simulink model "pv_and_wind_completed"  (R2018a)
settings: Solver=VariableStepAuto  StartTime=0.0  StopTime=2.4  RelTol=1e-3
libraries: powerlib x50, powerlib_meascontrol x12, simulink x10, re_lib x2, peGeneralControl x1, simulink_extras x1
(part 1 of 2)
settings SolverCC: AlgebraicLoopSolver=LineSearch

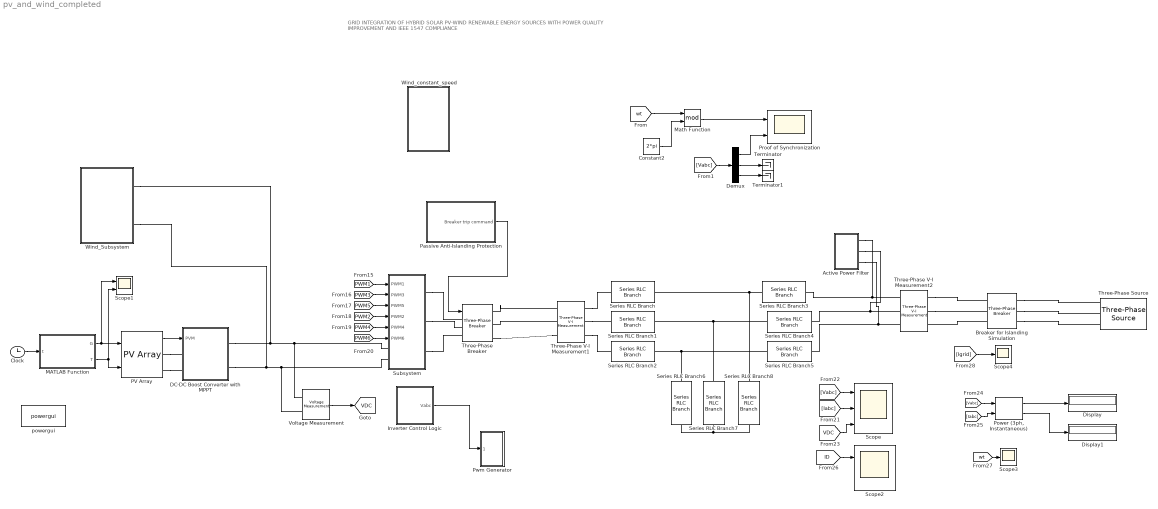
== system pv_and_wind_completed ==
  note: GRID INTEGRATION OF HYBRID SOLAR PV-WIND RENEWABLE ENERGY SOURCES WITH POWER QUALITY IMPROVEMENT AND IEEE 1547 COMPLIANCE
  Active Power Filter : Subsystem
  Breaker for Islanding Simulation : powerlib/Elements/Three-Phase Breaker  InitialState=closed  SwitchA=on  SwitchB=on  SwitchC=on  SwitchTimes=[9999]  External=off  BreakerResistance=0.01  SnubberResistance=1e6  SnubberCapacitance=inf  Measurements=None
  Clock : Clock
  Constant2 : Constant  Value=2*pi
  DC-DC Boost Converter with MPPT : Subsystem
  Demux : Demux  Outputs=3
  Display : Display
  Display1 : Display
  Inverter Control Logic : Subsystem
  MATLAB Function : MATLAB Function  TreatAsAtomicUnit=on
  Math Function : Math  Operator=mod  SaturateOnIntegerOverflow=on
  PV Array : re_lib/Solar/PV Array  Npar=40  Nser=10  PlotType=array @ 1000 W/m2 & specified temperatures  S_vec="[ 1000  500  100 ]"  Temp_C_vec="[ 45 25  ]"  ModuleName=1Soltech 1STH-215-P  PlotWhenSelected=off  Pm=213.15  Ncell=60  Voc=36.3  Isc=7.84  Vm=29  Im=7.35  beta_Voc_pc=-0.36099  alpha_Isc_pc=0.102  beta_Voc=-0.13104  alpha_Isc=0.007997  IL=7.8649  I0=2.9259e-10  nI=0.98117  Rsh=313.3991  Rs=0.39383  BAL=off  Tc=1e-6  Tfilter=5e-5
  Passive Anti-Islanding Protection : Subsystem
  "Power (3ph, Instantaneous)" : powerlib_meascontrol/Measurements/Power (3ph, Instantaneous)
      settings: SourceProductName=Simscape Power Systems
  Proof of Synchronization : Scope  NumInputPorts=2
  "Pwm Generator " : Subsystem
  Scope : Scope  NumInputPorts=3
  Scope1 : Scope  NumInputPorts=2
  Scope2 : Scope  NumInputPorts=2
  Scope3 : Scope
  Scope4 : Scope
  Series RLC Branch : powerlib/Elements/Series RLC Branch  LConnTagsString=__new0  RConnTagsString=__new0  BranchType=RL  Resistance=1e-3  Inductance=1e-3  SetiL0=off  InitialCurrent=0  Capacitance=1e-6  Setx0=off  InitialVoltage=0  Measurements=None
  Series RLC Branch1 : powerlib/Elements/Series RLC Branch  LConnTagsString=__new0  RConnTagsString=__new0  BranchType=RL  Resistance=1e-3  Inductance=1e-3  SetiL0=off  InitialCurrent=0  Capacitance=1e-6  Setx0=off  InitialVoltage=0  Measurements=None
  Series RLC Branch2 : powerlib/Elements/Series RLC Branch  LConnTagsString=__new0  RConnTagsString=__new0  BranchType=RL  Resistance=1e-3  Inductance=1e-3  SetiL0=off  InitialCurrent=0  Capacitance=1e-6  Setx0=off  InitialVoltage=0  Measurements=None
  Series RLC Branch3 : powerlib/Elements/Series RLC Branch  LConnTagsString=__new0  RConnTagsString=__new0  BranchType=RL  Resistance=1e-3  Inductance=0.5e-3  SetiL0=on  InitialCurrent=10  Capacitance=1e-6  Setx0=off  InitialVoltage=0  Measurements=None
  Series RLC Branch4 : powerlib/Elements/Series RLC Branch  LConnTagsString=__new0  RConnTagsString=__new0  BranchType=RL  Resistance=1e-3  Inductance=0.5e-3  SetiL0=on  InitialCurrent=10  Capacitance=1e-6  Setx0=off  InitialVoltage=0  Measurements=None
  Series RLC Branch5 : powerlib/Elements/Series RLC Branch  LConnTagsString=__new0  RConnTagsString=__new0  BranchType=RL  Resistance=1e-3  Inductance=0.5e-3  SetiL0=on  InitialCurrent=10  Capacitance=1e-6  Setx0=off  InitialVoltage=0  Measurements=None
  Series RLC Branch6 : powerlib/Elements/Series RLC Branch  LConnTagsString=__new0  RConnTagsString=__new0  BranchType=RC  Resistance=1e-3  Inductance=1000e-3  SetiL0=off  InitialCurrent=0  Capacitance=100e-6  Setx0=off  InitialVoltage=0  Measurements=None
  Series RLC Branch7 : powerlib/Elements/Series RLC Branch  LConnTagsString=__new0  RConnTagsString=__new0  BranchType=RC  Resistance=1e-3  Inductance=1000e-3  SetiL0=off  InitialCurrent=0  Capacitance=100e-6  Setx0=off  InitialVoltage=0  Measurements=None
  Series RLC Branch8 : powerlib/Elements/Series RLC Branch  LConnTagsString=__new0  RConnTagsString=__new0  BranchType=RC  Resistance=1e-3  Inductance=1000e-3  SetiL0=off  InitialCurrent=0  Capacitance=100e-6  Setx0=off  InitialVoltage=0  Measurements=None
  Subsystem : Subsystem
  Terminator : Terminator
  Terminator1 : Terminator
  Three-Phase V-I Measurement1 : powerlib/Measurements/Three-Phase V-I Measurement  VoltageMeasurement=no  SetLabelV=off  LabelV=Vabc  Vpu=off  VpuLL=off  CurrentMeasurement=yes  SetLabelI=on  LabelI=Iabc  Ipu=off  Pbase=100e6  Vbase=500e3  OutputType=Complex  PhasorSimulation=off  PSBequivalent=0
  Three-Phase V-I Measurement2 : powerlib/Measurements/Three-Phase V-I Measurement  VoltageMeasurement=phase-to-ground  SetLabelV=on  LabelV=Vabc  Vpu=off  VpuLL=off  CurrentMeasurement=yes  SetLabelI=on  LabelI=Igrid  Ipu=off  Pbase=100e6  Vbase=500e3  OutputType=Complex  PhasorSimulation=off  PSBequivalent=0
  Three-Phase Breaker : powerlib/Elements/Three-Phase Breaker  InitialState=closed  SwitchA=on  SwitchB=on  SwitchC=on  SwitchTimes=[9999]  External=on  BreakerResistance=0.01  SnubberResistance=1e6  SnubberCapacitance=inf  Measurements=None
  Three-Phase Source : powerlib/Electrical Sources/Three-Phase Source  InternalConnection=Yg  VoltagePhases=off  Voltage=400  PhaseAngle=0  Voltage_phases=[25e3 25e3 25e3]/sqrt(3)  PhaseAngles_phases=[0 -120 +120]  Frequency=50  NonIdealSource=on  SpecifyImpedance=off  Resistance=1e-3  Inductance=1e-5  ShortCircuitLevel=10e-6  BaseVoltage=400  XRratio=7  BusType=swing  Pref=10e3  Qref=0  Prefabc=[10e3, 10e3, 10e3]  Qrefabc=[0, 0, 0]  Qmin=-inf  Qmax=inf
  Voltage Measurement : powerlib/Measurements/Voltage Measurement  PhasorSimulation=off  OutputType=Complex  PSBequivalent=0
  Wind_Subsystem : Subsystem
  "Wind_constant_speed " : Subsystem
  powergui : powerlib/powergui  Priority=1  SimulationMode=Discrete  SampleTime=1e-6  frequency=60  Iterations=50  frequencyindice=0  Pbase=100e6  ErrMax=1e-4  UnitsV=kV  UnitsW=MW  buscounter=0  FunctionMessages=off  echomessages=off  EnableUseOfTLC=off  CurrentSourceSwitches=off  DisableSnubberDevices=off  DisableRonSwitches=off  DisableVfSwitches=off  DisplayEquations=off  SolverType=Tustin/Backward Euler (TBE)  Interpol=off  ExternalGateDelay=off  methode=off  Ts=100  x0status=blocks  SPID=off  SwTol=0  HookPort=off  RestoreLinks=warning  ResistiveCurrentMeasurement=off  Frange=[0:2:500]  Ylog=off  Xlog=on  ShowGrid=off  save=off  variable=ZData  structure=Grid_current  ZoomFFT=off  StartTime=0.4  cycles=5  DisplayStyle=1  fundamental=50  FreqAxis=off  MaxFrequency=1000  frequencyindicesteady=1  RmsSteady=1  display=off
  tag scope: VDC=global
  wires:
  Voltage Measurement/1 -> [VDC]
  [PWM6] -> Subsystem/6(PWM6)
  [PWM1] -> Subsystem/1(PWM1)
  "Power (3ph, Instantaneous)"/1 -> Display/1
  PV Array/1 -> DC-DC Boost Converter with MPPT/1("PVM ")
  [Iabc] -> "Power (3ph, Instantaneous)"/2
  [PWM3] -> Subsystem/2(PWM3)
  [Igrid] -> Scope4/1
  Inverter Control Logic/1(Vabc) -> "Pwm Generator "/1(1)
  [PWM4] -> Subsystem/5(PWM4)
  [Vabc] -> Scope/1
  [Vabc] -> "Power (3ph, Instantaneous)"/1
  [ID] -> Scope2/1
  "Power (3ph, Instantaneous)"/2 -> Display1/1
  [wt] -> Scope3/1
  [PWM2] -> Subsystem/4(PWM2)
  [VDC] -> Scope/3
  [PWM5] -> Subsystem/3(PWM5)
  [Iabc] -> Scope/2
  Passive Anti-Islanding Protection/1("Breaker trip command ") -> Three-Phase Breaker/1
  Demux/1 -> Proof of Synchronization/2
  Demux/2 -> Terminator/1
  Constant2/1 -> Math Function/2
  [wt] -> Math Function/1
  Math Function/1 -> Proof of Synchronization/1
  [Vabc] -> Demux/1
  Demux/3 -> Terminator1/1
  MATLAB Function/1(G) -> Scope1/1, PV Array/1
  MATLAB Function/2(T) -> Scope1/2, PV Array/2
  Clock/1 -> MATLAB Function/1(t)
  connections:
  Series RLC Branch7/RConn1 -- Series RLC Branch8/RConn1 -- Series RLC Branch6/RConn1
  Series RLC Branch8/LConn1 -- Series RLC Branch/RConn1 -- Series RLC Branch3/LConn1
  Series RLC Branch7/LConn1 -- Series RLC Branch1/RConn1 -- Series RLC Branch4/LConn1
  Series RLC Branch6/LConn1 -- Series RLC Branch2/RConn1 -- Series RLC Branch5/LConn1
  PV Array/RConn1 -- DC-DC Boost Converter with MPPT/LConn1
  Series RLC Branch3/RConn1 -- Active Power Filter/RConn1 -- Three-Phase V-I Measurement2/RConn1
  Series RLC Branch4/RConn1 -- Active Power Filter/RConn2 -- Three-Phase V-I Measurement2/RConn2
  Three-Phase V-I Measurement1/RConn3 -- Series RLC Branch2/LConn1
  Three-Phase V-I Measurement1/RConn1 -- Series RLC Branch/LConn1
  PV Array/RConn2 -- DC-DC Boost Converter with MPPT/LConn2
  Three-Phase V-I Measurement1/RConn2 -- Series RLC Branch1/LConn1
  Series RLC Branch5/RConn1 -- Active Power Filter/RConn3 -- Three-Phase V-I Measurement2/RConn3
  DC-DC Boost Converter with MPPT/RConn1 -- Wind_Subsystem/RConn1 -- Subsystem/LConn1 -- Voltage Measurement/LConn1
  DC-DC Boost Converter with MPPT/RConn2 -- Wind_Subsystem/RConn2 -- Subsystem/LConn2 -- Voltage Measurement/LConn2
  Subsystem/RConn1 -- Three-Phase Breaker/LConn1
  Subsystem/RConn2 -- Three-Phase Breaker/LConn2
  Subsystem/RConn3 -- Three-Phase Breaker/LConn3
  Three-Phase Breaker/RConn1 -- Three-Phase V-I Measurement1/LConn1
  Three-Phase V-I Measurement1/LConn2 -- Three-Phase Breaker/RConn2
  Three-Phase Breaker/RConn3 -- Three-Phase V-I Measurement1/LConn3
  Three-Phase V-I Measurement2/LConn1 -- Breaker for Islanding Simulation/LConn1
  Three-Phase V-I Measurement2/LConn2 -- Breaker for Islanding Simulation/LConn2
  Breaker for Islanding Simulation/LConn3 -- Three-Phase V-I Measurement2/LConn3
  Breaker for Islanding Simulation/RConn1 -- Three-Phase Source/RConn1
  Breaker for Islanding Simulation/RConn2 -- Three-Phase Source/RConn2
  Breaker for Islanding Simulation/RConn3 -- Three-Phase Source/RConn3

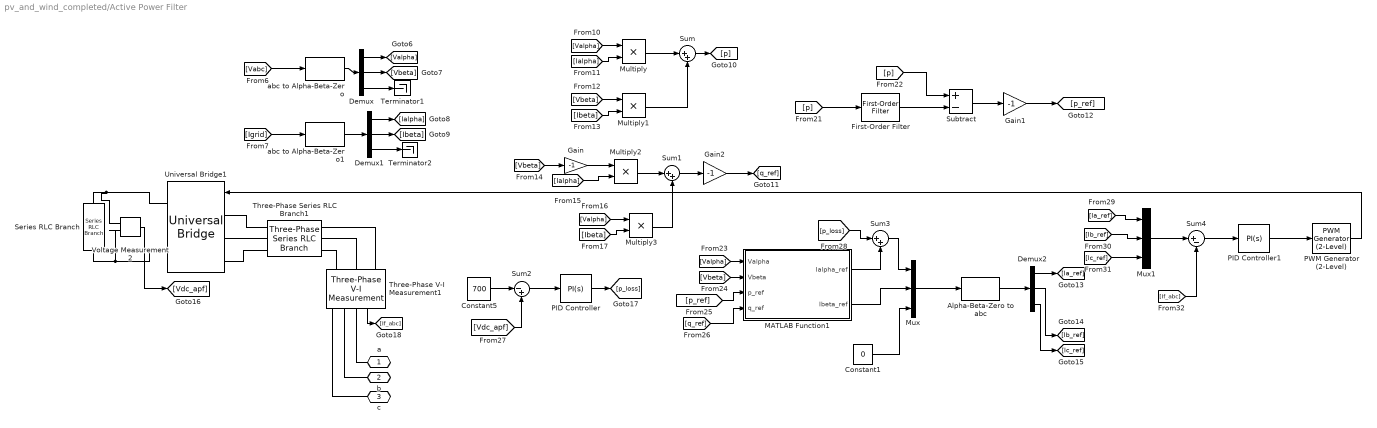
== system pv_and_wind_completed/Active Power Filter ==
  Alpha-Beta-Zero to abc : powerlib_meascontrol/Transformations/Alpha-Beta-Zero to abc
      settings: SourceProductName=Simscape Power Systems  SourceProductBaseCode=PS
  Constant1 : Constant  Value=0
  Constant5 : Constant  Value=700
  Demux : Demux  Outputs=3
  Demux1 : Demux  Outputs=3
  Demux2 : Demux  Outputs=3
  First-Order Filter : powerlib_meascontrol/Filters/First-Order Filter  FilterType=Lowpass  Tc=0.03183  Ts=0  Initialize=on  Vac_Init=[0, 0, 50]  Vdc_Init=0  PlotResponse=off  FreqRange="[0,  200,  1]"
      settings: SourceProductName=Simscape Power Systems
  Gain : Gain  Gain=-1
  Gain1 : Gain  Gain=-1
  Gain2 : Gain  Gain=-1
  MATLAB Function1 : MATLAB Function  TreatAsAtomicUnit=on
  Multiply{,1..3} (4 alike) : Product
  Mux : Mux  Inputs=3
  Mux1 : Mux  Inputs=3
  PID Controller : simulink/Continuous/PID Controller  Controller=PI  TimeDomain=Continuous-time  SampleTime=-1  IntegratorMethod=Forward Euler  FilterMethod=Forward Euler  Form=Parallel  UseFilter=on  ControllerParametersSource=internal  P=1  I=1  D=0  N=100  InitialConditionSource=internal  InitialConditionForIntegrator=0  InitialConditionForFilter=0  ExternalReset=none  LimitOutput=off  UpperSaturationLimit=inf  LowerSaturationLimit=-inf  LinearizeAsGain=on  AntiWindupMode=none  Kb=1  TrackingMode=off  Kt=1  PParamMin=[]  PParamMax=[]  IParamMin=[]  IParamMax=[]  DParamMin=[]  DParamMax=[]  NParamMin=[]  NParamMax=[]  KbParamMin=[]  KbParamMax=[]  KtParamMin=[]  KtParamMax=[]  POutMin=[]  POutMax=[]  IOutMin=[]  IOutMax=[]  DOutMin=[]  DOutMax=[]  NOutMin=[]  NOutMax=[]  KbOutMin=[]  KbOutMax=[]  KtOutMin=[]  KtOutMax=[]  IntegratorOutMin=[]  IntegratorOutMax=[]  FilterOutMin=[]  FilterOutMax=[]  SumOutMin=[]  SumOutMax=[]  SumI1OutMin=[]  SumI1OutMax=[]  SumI2OutMin=[]  SumI2OutMax=[]  SumI3OutMin=[]  SumI3OutMax=[]  SumDOutMin=[]  SumDOutMax=[]  SaturationOutMin=[]  SaturationOutMax=[]  IntegratorContinuousStateAttributes=''  IntegratorStateMustResolveToSignalObject=off  IntegratorRTWStateStorageClass=Auto  FilterContinuousStateAttributes=''  FilterStateMustResolveToSignalObject=off  FilterRTWStateStorageClass=Auto  DifferentiatorICPrevScaledInput=0  DifferentiatorOutMin=[]  DifferentiatorOutMax=[]  FilterDiffOutCoefMin=[]  FilterDiffOutCoefMax=[]  SumDenOutMin=[]  SumDenOutMax=[]  SumNumOutMin=[]  SumNumOutMax=[]  ReciprocalOutMin=[]  ReciprocalOutMax=[]  DivideOutMin=[]  DivideOutMax=[]  TunerSelectOption=Transfer Function Based (PID Tuner App)
  PID Controller1 : simulink/Continuous/PID Controller  Controller=PI  TimeDomain=Continuous-time  SampleTime=-1  IntegratorMethod=Forward Euler  FilterMethod=Forward Euler  Form=Parallel  UseFilter=on  ControllerParametersSource=internal  P=50  I=1000  D=0  N=100  InitialConditionSource=internal  InitialConditionForIntegrator=0  InitialConditionForFilter=0  ExternalReset=none  LimitOutput=off  UpperSaturationLimit=inf  LowerSaturationLimit=-inf  LinearizeAsGain=on  AntiWindupMode=none  Kb=1  TrackingMode=off  Kt=1  PParamMin=[]  PParamMax=[]  IParamMin=[]  IParamMax=[]  DParamMin=[]  DParamMax=[]  NParamMin=[]  NParamMax=[]  KbParamMin=[]  KbParamMax=[]  KtParamMin=[]  KtParamMax=[]  POutMin=[]  POutMax=[]  IOutMin=[]  IOutMax=[]  DOutMin=[]  DOutMax=[]  NOutMin=[]  NOutMax=[]  KbOutMin=[]  KbOutMax=[]  KtOutMin=[]  KtOutMax=[]  IntegratorOutMin=[]  IntegratorOutMax=[]  FilterOutMin=[]  FilterOutMax=[]  SumOutMin=[]  SumOutMax=[]  SumI1OutMin=[]  SumI1OutMax=[]  SumI2OutMin=[]  SumI2OutMax=[]  SumI3OutMin=[]  SumI3OutMax=[]  SumDOutMin=[]  SumDOutMax=[]  SaturationOutMin=[]  SaturationOutMax=[]  IntegratorContinuousStateAttributes=''  IntegratorStateMustResolveToSignalObject=off  IntegratorRTWStateStorageClass=Auto  FilterContinuousStateAttributes=''  FilterStateMustResolveToSignalObject=off  FilterRTWStateStorageClass=Auto  DifferentiatorICPrevScaledInput=0  DifferentiatorOutMin=[]  DifferentiatorOutMax=[]  FilterDiffOutCoefMin=[]  FilterDiffOutCoefMax=[]  SumDenOutMin=[]  SumDenOutMax=[]  SumNumOutMin=[]  SumNumOutMax=[]  ReciprocalOutMin=[]  ReciprocalOutMax=[]  DivideOutMin=[]  DivideOutMax=[]  TunerSelectOption=Transfer Function Based (PID Tuner App)
  PWM Generator (2-Level) : powerlib_meascontrol/Pulse & Signal Generators/PWM Generator (2-Level)  ModulatorType=Three-phase bridge (6 pulses)  ModulatorMode=Unsynchronized  Fc=10000  Pc=90  nF=27  MinMax="[ -1  1 ]"  SamplingTechnique=Natural  ModulatingSignals=off  m=0.8  Freq=60  Phase=0  Ts=0  ShowCarrierOutport=off
      settings: SourceProductName=Simscape Power Systems
  Series RLC Branch : powerlib/Elements/Series RLC Branch  LConnTagsString=__new0  RConnTagsString=__new0  BranchType=C  Resistance=1  Inductance=1e-3  SetiL0=off  InitialCurrent=0  Capacitance=2200e-6  Setx0=on  InitialVoltage=700  Measurements=None
  Subtract : Sum  Inputs=+-
  Sum : Sum  Inputs=|++
  Sum1 : Sum  Inputs=|++
  Sum2 : Sum  Inputs=|-+
  Sum3 : Sum  Inputs=|++
  Sum4 : Sum  Inputs=|+-
  Terminator1 : Terminator
  Terminator2 : Terminator
  Three-Phase Series RLC Branch1 : powerlib/Elements/Three-Phase Series RLC Branch  LConnTagsString=A|B|C  RConnTagsString=A|B|C  BranchType=RL  Resistance=0.1  Inductance=4e-3  Capacitance=1e-6  Measurements=None
  Three-Phase V-I Measurement1 : powerlib/Measurements/Three-Phase V-I Measurement  VoltageMeasurement=phase-to-ground  SetLabelV=off  LabelV=Vabc  Vpu=off  VpuLL=off  CurrentMeasurement=yes  SetLabelI=off  LabelI=Iabc  Ipu=off  Pbase=100e6  Vbase=500e3  OutputType=Complex  PhasorSimulation=off  PSBequivalent=0
  Universal Bridge1 : powerlib/Power Electronics/Universal Bridge  Arms=3  SnubberResistance=1e5  SnubberCapacitance=inf  Device=IGBT / Diodes  Ron=1e-3  Lon=0  ForwardVoltages="[  0  0  ]"  ForwardVoltage=0  GTOparameters=[ 10e-6 , 20e-6 ]  IGBTparameters=[ 1e-6 , 2e-6 ]  Measurements=None  Measurements_2=None  converterType=Rectifier
  Voltage Measurement2 : powerlib/Measurements/Voltage Measurement  PhasorSimulation=off  OutputType=Complex  PSBequivalent=0
  abc to Alpha-Beta-Zero : powerlib_meascontrol/Transformations/abc to Alpha-Beta-Zero
      settings: SourceProductName=Simscape Power Systems
  abc to Alpha-Beta-Zero1 : powerlib_meascontrol/Transformations/abc to Alpha-Beta-Zero
      settings: SourceProductName=Simscape Power Systems
  a : PMIOPort  Side=Right
  b : PMIOPort  Port=2  Side=Right
  c : PMIOPort  Port=3  Side=Right
  wires:
  Demux/3 -> Terminator1/1
  Subtract/1 -> Gain1/1
  [Igrid] -> abc to Alpha-Beta-Zero1/1
  [Ibeta] -> Multiply3/2
  Sum4/1 -> PID Controller1/1
  [Ic_ref] -> Mux1/3
  Sum1/1 -> Gain2/1
  MATLAB Function1/2(Ibeta_ref) -> Mux/2
  Gain1/1 -> [p_ref]
  [Vabc] -> abc to Alpha-Beta-Zero/1
  [p] -> Subtract/1
  Gain2/1 -> [q_ref]
  PID Controller1/1 -> PWM Generator (2-Level)/1
  Voltage Measurement2/1 -> [Vdc_apf]
  [Ialpha] -> Multiply/2
  Demux/2 -> [Vbeta]
  Multiply2/1 -> Sum1/1
  Alpha-Beta-Zero to abc/1 -> Demux2/1
  Multiply1/1 -> Sum/2
  [Vbeta] -> Multiply1/1
  Constant5/1 -> Sum2/1
  [If_abc] -> Sum4/2
  [Valpha] -> MATLAB Function1/1(Valpha)
  Sum/1 -> [p]
  [q_ref] -> MATLAB Function1/4(q_ref)
  Mux/1 -> Alpha-Beta-Zero to abc/1
  Demux2/3 -> [Ic_ref]
  [Vbeta] -> MATLAB Function1/2(Vbeta)
  [Valpha] -> Multiply/1
  Demux2/2 -> [Ib_ref]
  [Vdc_apf] -> Sum2/2
  [Vbeta] -> Gain/1
  [Ialpha] -> Multiply2/2
  Sum3/1 -> Mux/1
  Mux1/1 -> Sum4/1
  Demux2/1 -> [Ia_ref]
  [p_ref] -> MATLAB Function1/3(p_ref)
  Demux1/2 -> [Ibeta]
  Constant1/1 -> Mux/3
  abc to Alpha-Beta-Zero/1 -> Demux/1
  Three-Phase V-I Measurement1/2 -> [If_abc]
  PID Controller/1 -> [p_loss]
  [p_loss] -> Sum3/1
  MATLAB Function1/1(Ialpha_ref) -> Sum3/2
  [Valpha] -> Multiply3/1
  Sum2/1 -> PID Controller/1
  Gain/1 -> Multiply2/1
  [Ia_ref] -> Mux1/1
  abc to Alpha-Beta-Zero1/1 -> Demux1/1
  Demux1/1 -> [Ialpha]
  [Ibeta] -> Multiply1/2
  Multiply/1 -> Sum/1
  Demux/1 -> [Valpha]
  First-Order Filter/1 -> Subtract/2
  [Ib_ref] -> Mux1/2
  [p] -> First-Order Filter/1
  Multiply3/1 -> Sum1/2
  PWM Generator (2-Level)/1 -> Universal Bridge1/1
  Demux1/3 -> Terminator2/1
  connections:
  Three-Phase Series RLC Branch1/LConn2 -- Universal Bridge1/LConn2
  Series RLC Branch/LConn1 -- Voltage Measurement2/LConn1 -- Universal Bridge1/RConn1
  Universal Bridge1/LConn3 -- Three-Phase Series RLC Branch1/LConn3
  Three-Phase Series RLC Branch1/LConn1 -- Universal Bridge1/LConn1
  Series RLC Branch/RConn1 -- Voltage Measurement2/LConn2 -- Universal Bridge1/RConn2
  Three-Phase Series RLC Branch1/RConn1 -- Three-Phase V-I Measurement1/LConn1
  Three-Phase Series RLC Branch1/RConn3 -- Three-Phase V-I Measurement1/LConn3
  Three-Phase Series RLC Branch1/RConn2 -- Three-Phase V-I Measurement1/LConn2
  b/RConn1 -- Three-Phase V-I Measurement1/RConn2
  a/RConn1 -- Three-Phase V-I Measurement1/RConn1
  c/RConn1 -- Three-Phase V-I Measurement1/RConn3

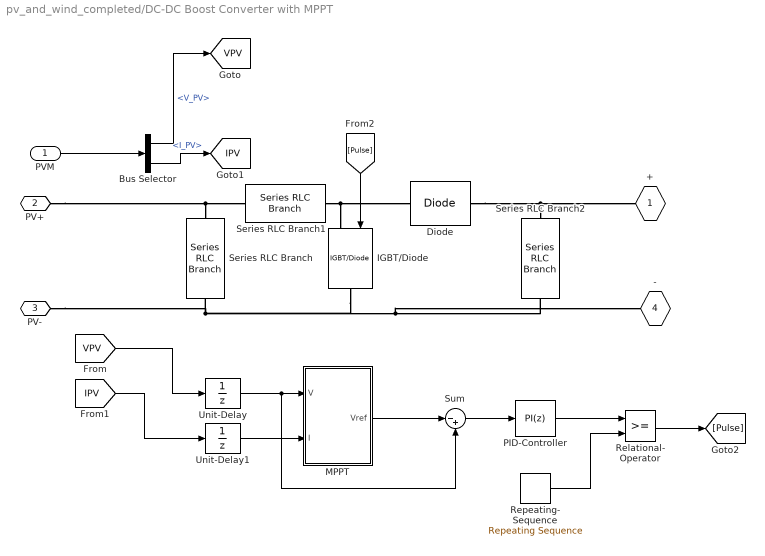
== system pv_and_wind_completed/DC-DC Boost Converter with MPPT ==
  "PVM " : Inport
  Bus Selector : BusSelector  OutputSignals=V_PV,I_PV
  Diode : powerlib/Power Electronics/Diode  Ron=0.001  Lon=0  Vf=0.8  IC=0  UseSnubber=0  Rs=500  Cs=250e-9  Measurements=off
  IGBT/Diode : powerlib/Power Electronics/IGBT//Diode  Ron=1e-3  Rs=1e5  Cs=inf  Measurements=off
  MPPT : MATLAB Function  TreatAsAtomicUnit=on
  PID-Controller : simulink/Continuous/PID Controller  Controller=PI  TimeDomain=Discrete-time  SampleTime=1e-3  IntegratorMethod=Forward Euler  FilterMethod=Forward Euler  Form=Parallel  UseFilter=on  ControllerParametersSource=internal  P=0.001  I=0.01  D=0  N=100  InitialConditionSource=internal  InitialConditionForIntegrator=0  InitialConditionForFilter=0  ExternalReset=none  LimitOutput=on  UpperSaturationLimit=0.95  LowerSaturationLimit=0  LinearizeAsGain=on  AntiWindupMode=none  Kb=1  TrackingMode=off  Kt=1  PParamMin=[]  PParamMax=[]  IParamMin=[]  IParamMax=[]  DParamMin=[]  DParamMax=[]  NParamMin=[]  NParamMax=[]  KbParamMin=[]  KbParamMax=[]  KtParamMin=[]  KtParamMax=[]  POutMin=[]  POutMax=[]  IOutMin=[]  IOutMax=[]  DOutMin=[]  DOutMax=[]  NOutMin=[]  NOutMax=[]  KbOutMin=[]  KbOutMax=[]  KtOutMin=[]  KtOutMax=[]  IntegratorOutMin=[]  IntegratorOutMax=[]  FilterOutMin=[]  FilterOutMax=[]  SumOutMin=[]  SumOutMax=[]  SumI1OutMin=[]  SumI1OutMax=[]  SumI2OutMin=[]  SumI2OutMax=[]  SumI3OutMin=[]  SumI3OutMax=[]  SumDOutMin=[]  SumDOutMax=[]  SaturationOutMin=[]  SaturationOutMax=[]  IntegratorContinuousStateAttributes=''  IntegratorStateMustResolveToSignalObject=off  IntegratorRTWStateStorageClass=Auto  FilterContinuousStateAttributes=''  FilterStateMustResolveToSignalObject=off  FilterRTWStateStorageClass=Auto  DifferentiatorICPrevScaledInput=0  DifferentiatorOutMin=[]  DifferentiatorOutMax=[]  FilterDiffOutCoefMin=[]  FilterDiffOutCoefMax=[]  SumDenOutMin=[]  SumDenOutMax=[]  SumNumOutMin=[]  SumNumOutMax=[]  ReciprocalOutMin=[]  ReciprocalOutMax=[]  DivideOutMin=[]  DivideOutMax=[]  TunerSelectOption=Transfer Function Based (PID Tuner App)
  Relational- Operator : RelationalOperator  OutDataTypeStr=boolean  RndMeth=Simplest
  Repeating- Sequence : simulink/Sources/Repeating Sequence  rep_seq_t=[0 0.0002]  rep_seq_y=[0 1]
  Series RLC Branch : powerlib/Elements/Series RLC Branch  LConnTagsString=__new0  RConnTagsString=__new0  BranchType=RC  Resistance=1e-3  Inductance=1e-3  SetiL0=off  InitialCurrent=0  Capacitance=1000e-6  Setx0=off  InitialVoltage=0  Measurements=None
  Series RLC Branch1 : powerlib/Elements/Series RLC Branch  LConnTagsString=__new0  RConnTagsString=__new0  BranchType=L  Resistance=1e-3  Inductance=1.5e-3  SetiL0=off  InitialCurrent=0  Capacitance=1000e-6  Setx0=off  InitialVoltage=0  Measurements=None
  Series RLC Branch2 : powerlib/Elements/Series RLC Branch  LConnTagsString=__new0  RConnTagsString=__new0  BranchType=C  Resistance=1e-3  Inductance=1e-3  SetiL0=off  InitialCurrent=0  Capacitance=3227e-6  Setx0=on  InitialVoltage=400  Measurements=None
  Sum : Sum  Inputs=|-+
  Unit-Delay : UnitDelay  SampleTime=1e-4
  Unit-Delay1 : UnitDelay  SampleTime=1e-4
  + : PMIOPort  Side=Right
  PV+ : PMIOPort  Port=2  Side=Left
  PV- : PMIOPort  Port=3  Side=Left
  - : PMIOPort  Port=4  Side=Right
  tag scope: IPV=global, VPV=global
  wires:
  [Pulse] -> IGBT/Diode/1
  Bus Selector/1 -> [VPV]  "<V_PV>"
  Bus Selector/2 -> [IPV]  "<I_PV>"
  "PVM "/1 -> Bus Selector/1
  MPPT/1(Vref) -> Sum/1
  [VPV] -> Unit-Delay/1
  Relational- Operator/1 -> [Pulse]
  Unit-Delay/1 -> Sum/2, MPPT/1(V)
  Repeating- Sequence/1 -> Relational- Operator/2
  PID-Controller/1 -> Relational- Operator/1
  Unit-Delay1/1 -> MPPT/2(I)
  Sum/1 -> PID-Controller/1
  [IPV] -> Unit-Delay1/1
  connections:
  Diode/RConn1 -- +/RConn1 -- Series RLC Branch2/LConn1
  Series RLC Branch/RConn1 -- PV-/RConn1 -- -/RConn1 -- Series RLC Branch2/RConn1 -- IGBT/Diode/RConn1
  Series RLC Branch1/LConn1 -- Diode/LConn1 -- IGBT/Diode/LConn1
  Series RLC Branch/LConn1 -- PV+/RConn1 -- Series RLC Branch1/RConn1

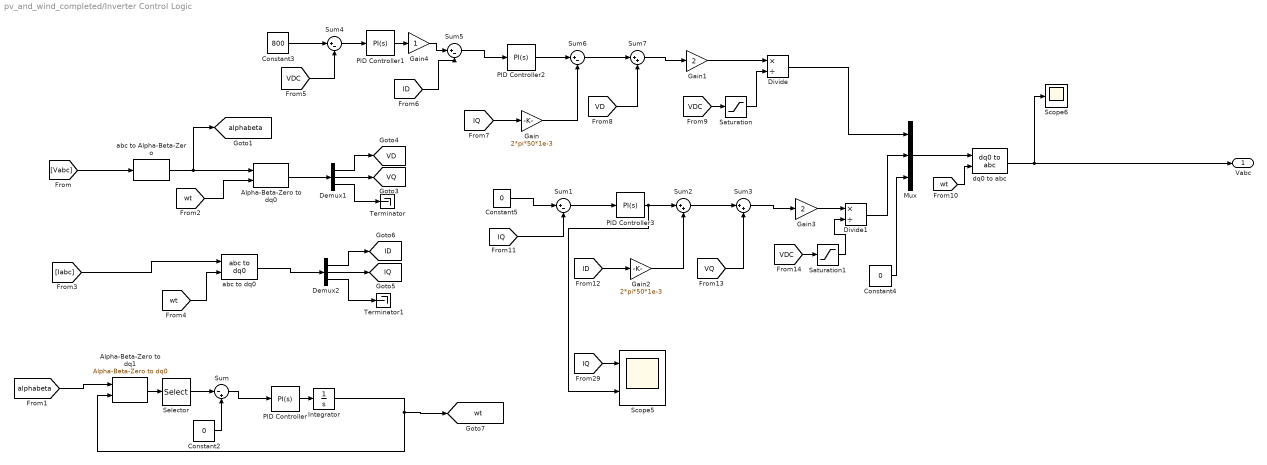
== system pv_and_wind_completed/Inverter Control Logic ==
  Alpha-Beta-Zero to dq0 : powerlib_meascontrol/Transformations/Alpha-Beta-Zero to dq0  Alignment=90 degrees behind phase A axis
      settings: SourceProductName=Simscape Power Systems
  Alpha-Beta-Zero to dq1 : powerlib_meascontrol/Transformations/Alpha-Beta-Zero to dq0  Alignment=90 degrees behind phase A axis
      settings: SourceProductName=Simscape Power Systems
  Constant2 : Constant  Value=0
  Constant3 : Constant  Value=800
  Constant4 : Constant  Value=0
  Constant5 : Constant  Value=0
  Demux1 : Demux  Outputs=3
  Demux2 : Demux  Outputs=3
  Divide : Product  Inputs=*/
  Divide1 : Product  Inputs=*/
  Gain : Gain  Gain=2*pi*50*1e-3
  Gain1 : Gain  Gain=2
  Gain2 : Gain  Gain=2*pi*50*1e-3
  Gain3 : Gain  Gain=2
  Gain4 : Gain
  Integrator : Integrator
  Mux : Mux  Inputs=3
  PID Controller : simulink/Continuous/PID Controller  Controller=PI  TimeDomain=Continuous-time  SampleTime=-1  IntegratorMethod=Forward Euler  FilterMethod=Forward Euler  Form=Parallel  UseFilter=on  ControllerParametersSource=internal  P=10  I=50000  D=0  N=100  InitialConditionSource=internal  InitialConditionForIntegrator=0  InitialConditionForFilter=0  ExternalReset=none  LimitOutput=off  UpperSaturationLimit=inf  LowerSaturationLimit=-inf  LinearizeAsGain=on  AntiWindupMode=none  Kb=1  TrackingMode=off  Kt=1  PParamMin=[]  PParamMax=[]  IParamMin=[]  IParamMax=[]  DParamMin=[]  DParamMax=[]  NParamMin=[]  NParamMax=[]  KbParamMin=[]  KbParamMax=[]  KtParamMin=[]  KtParamMax=[]  POutMin=[]  POutMax=[]  IOutMin=[]  IOutMax=[]  DOutMin=[]  DOutMax=[]  NOutMin=[]  NOutMax=[]  KbOutMin=[]  KbOutMax=[]  KtOutMin=[]  KtOutMax=[]  IntegratorOutMin=[]  IntegratorOutMax=[]  FilterOutMin=[]  FilterOutMax=[]  SumOutMin=[]  SumOutMax=[]  SumI1OutMin=[]  SumI1OutMax=[]  SumI2OutMin=[]  SumI2OutMax=[]  SumI3OutMin=[]  SumI3OutMax=[]  SumDOutMin=[]  SumDOutMax=[]  SaturationOutMin=[]  SaturationOutMax=[]  IntegratorContinuousStateAttributes=''  IntegratorStateMustResolveToSignalObject=off  IntegratorRTWStateStorageClass=Auto  FilterContinuousStateAttributes=''  FilterStateMustResolveToSignalObject=off  FilterRTWStateStorageClass=Auto  DifferentiatorICPrevScaledInput=0  DifferentiatorOutMin=[]  DifferentiatorOutMax=[]  FilterDiffOutCoefMin=[]  FilterDiffOutCoefMax=[]  SumDenOutMin=[]  SumDenOutMax=[]  SumNumOutMin=[]  SumNumOutMax=[]  ReciprocalOutMin=[]  ReciprocalOutMax=[]  DivideOutMin=[]  DivideOutMax=[]  TunerSelectOption=Transfer Function Based (PID Tuner App)
  PID Controller1 : simulink/Continuous/PID Controller  Controller=PI  TimeDomain=Continuous-time  SampleTime=-1  IntegratorMethod=Forward Euler  FilterMethod=Forward Euler  Form=Parallel  UseFilter=on  ControllerParametersSource=internal  P=0.5  I=10  D=0  N=100  InitialConditionSource=internal  InitialConditionForIntegrator=0  InitialConditionForFilter=0  ExternalReset=none  LimitOutput=on  UpperSaturationLimit=400  LowerSaturationLimit=-400  LinearizeAsGain=on  AntiWindupMode=none  Kb=1  TrackingMode=off  Kt=1  PParamMin=[]  PParamMax=[]  IParamMin=[]  IParamMax=[]  DParamMin=[]  DParamMax=[]  NParamMin=[]  NParamMax=[]  KbParamMin=[]  KbParamMax=[]  KtParamMin=[]  KtParamMax=[]  POutMin=[]  POutMax=[]  IOutMin=[]  IOutMax=[]  DOutMin=[]  DOutMax=[]  NOutMin=[]  NOutMax=[]  KbOutMin=[]  KbOutMax=[]  KtOutMin=[]  KtOutMax=[]  IntegratorOutMin=[]  IntegratorOutMax=[]  FilterOutMin=[]  FilterOutMax=[]  SumOutMin=[]  SumOutMax=[]  SumI1OutMin=[]  SumI1OutMax=[]  SumI2OutMin=[]  SumI2OutMax=[]  SumI3OutMin=[]  SumI3OutMax=[]  SumDOutMin=[]  SumDOutMax=[]  SaturationOutMin=[]  SaturationOutMax=[]  IntegratorContinuousStateAttributes=''  IntegratorStateMustResolveToSignalObject=off  IntegratorRTWStateStorageClass=Auto  FilterContinuousStateAttributes=''  FilterStateMustResolveToSignalObject=off  FilterRTWStateStorageClass=Auto  DifferentiatorICPrevScaledInput=0  DifferentiatorOutMin=[]  DifferentiatorOutMax=[]  FilterDiffOutCoefMin=[]  FilterDiffOutCoefMax=[]  SumDenOutMin=[]  SumDenOutMax=[]  SumNumOutMin=[]  SumNumOutMax=[]  ReciprocalOutMin=[]  ReciprocalOutMax=[]  DivideOutMin=[]  DivideOutMax=[]  TunerSelectOption=Transfer Function Based (PID Tuner App)
  PID Controller2 : simulink/Continuous/PID Controller  Controller=PI  TimeDomain=Continuous-time  SampleTime=-1  IntegratorMethod=Forward Euler  FilterMethod=Forward Euler  Form=Parallel  UseFilter=on  ControllerParametersSource=internal  P=1  I=1  D=0  N=100  InitialConditionSource=internal  InitialConditionForIntegrator=0  InitialConditionForFilter=0  ExternalReset=none  LimitOutput=on  UpperSaturationLimit=400  LowerSaturationLimit=-400  LinearizeAsGain=on  AntiWindupMode=none  Kb=1  TrackingMode=off  Kt=1  PParamMin=[]  PParamMax=[]  IParamMin=[]  IParamMax=[]  DParamMin=[]  DParamMax=[]  NParamMin=[]  NParamMax=[]  KbParamMin=[]  KbParamMax=[]  KtParamMin=[]  KtParamMax=[]  POutMin=[]  POutMax=[]  IOutMin=[]  IOutMax=[]  DOutMin=[]  DOutMax=[]  NOutMin=[]  NOutMax=[]  KbOutMin=[]  KbOutMax=[]  KtOutMin=[]  KtOutMax=[]  IntegratorOutMin=[]  IntegratorOutMax=[]  FilterOutMin=[]  FilterOutMax=[]  SumOutMin=[]  SumOutMax=[]  SumI1OutMin=[]  SumI1OutMax=[]  SumI2OutMin=[]  SumI2OutMax=[]  SumI3OutMin=[]  SumI3OutMax=[]  SumDOutMin=[]  SumDOutMax=[]  SaturationOutMin=[]  SaturationOutMax=[]  IntegratorContinuousStateAttributes=''  IntegratorStateMustResolveToSignalObject=off  IntegratorRTWStateStorageClass=Auto  FilterContinuousStateAttributes=''  FilterStateMustResolveToSignalObject=off  FilterRTWStateStorageClass=Auto  DifferentiatorICPrevScaledInput=0  DifferentiatorOutMin=[]  DifferentiatorOutMax=[]  FilterDiffOutCoefMin=[]  FilterDiffOutCoefMax=[]  SumDenOutMin=[]  SumDenOutMax=[]  SumNumOutMin=[]  SumNumOutMax=[]  ReciprocalOutMin=[]  ReciprocalOutMax=[]  DivideOutMin=[]  DivideOutMax=[]  TunerSelectOption=Transfer Function Based (PID Tuner App)
  PID Controller3 : simulink/Continuous/PID Controller  Controller=PI  TimeDomain=Continuous-time  SampleTime=-1  IntegratorMethod=Forward Euler  FilterMethod=Forward Euler  Form=Parallel  UseFilter=on  ControllerParametersSource=internal  P=1  I=1  D=0  N=100  InitialConditionSource=internal  InitialConditionForIntegrator=0  InitialConditionForFilter=0  ExternalReset=none  LimitOutput=off  UpperSaturationLimit=inf  LowerSaturationLimit=-inf  LinearizeAsGain=on  AntiWindupMode=none  Kb=1  TrackingMode=off  Kt=1  PParamMin=[]  PParamMax=[]  IParamMin=[]  IParamMax=[]  DParamMin=[]  DParamMax=[]  NParamMin=[]  NParamMax=[]  KbParamMin=[]  KbParamMax=[]  KtParamMin=[]  KtParamMax=[]  POutMin=[]  POutMax=[]  IOutMin=[]  IOutMax=[]  DOutMin=[]  DOutMax=[]  NOutMin=[]  NOutMax=[]  KbOutMin=[]  KbOutMax=[]  KtOutMin=[]  KtOutMax=[]  IntegratorOutMin=[]  IntegratorOutMax=[]  FilterOutMin=[]  FilterOutMax=[]  SumOutMin=[]  SumOutMax=[]  SumI1OutMin=[]  SumI1OutMax=[]  SumI2OutMin=[]  SumI2OutMax=[]  SumI3OutMin=[]  SumI3OutMax=[]  SumDOutMin=[]  SumDOutMax=[]  SaturationOutMin=[]  SaturationOutMax=[]  IntegratorContinuousStateAttributes=''  IntegratorStateMustResolveToSignalObject=off  IntegratorRTWStateStorageClass=Auto  FilterContinuousStateAttributes=''  FilterStateMustResolveToSignalObject=off  FilterRTWStateStorageClass=Auto  DifferentiatorICPrevScaledInput=0  DifferentiatorOutMin=[]  DifferentiatorOutMax=[]  FilterDiffOutCoefMin=[]  FilterDiffOutCoefMax=[]  SumDenOutMin=[]  SumDenOutMax=[]  SumNumOutMin=[]  SumNumOutMax=[]  ReciprocalOutMin=[]  ReciprocalOutMax=[]  DivideOutMin=[]  DivideOutMax=[]  TunerSelectOption=Transfer Function Based (PID Tuner App)
  Saturation : Saturate  UpperLimit=1500  LowerLimit=50
  Saturation1 : Saturate  UpperLimit=1500  LowerLimit=50
  Scope5 : Scope  NumInputPorts=2
  Scope6 : Scope
  Selector : Selector  InputPortWidth=3  IndexOptions=Index vector (dialog)  Indices=2  OutputSizes=1
  Sum : Sum  Inputs=|-+
  Sum{1,4..6} (4 alike) : Sum  Inputs=|+-
  Sum2 : Sum  Inputs=|++
  Sum3 : Sum  Inputs=|++
  Sum7 : Sum  Inputs=|++
  Terminator : Terminator
  Terminator1 : Terminator
  abc to Alpha-Beta-Zero : powerlib_meascontrol/Transformations/abc to Alpha-Beta-Zero
      settings: SourceProductName=Simscape Power Systems
  abc to dq0 : powerlib_meascontrol/Transformations/abc to dq0  Alignment=90 degrees behind phase A axis
  dq0 to abc : powerlib_meascontrol/Transformations/dq0 to abc  Alignment=90 degrees behind phase A axis
  Vabc : Outport
  tag scope: ID=global, IQ=global, VD=global, VQ=global, alphabeta=global, wt=global
  wires:
  Demux1/2 -> [VQ]
  Sum4/1 -> PID Controller1/1
  Constant3/1 -> Sum4/1
  Mux/1 -> dq0 to abc/1
  Sum5/1 -> PID Controller2/1
  Sum2/1 -> Sum3/1
  PID Controller3/1 -> Scope5/2, Sum2/1
  [alphabeta] -> Alpha-Beta-Zero to dq1/1
  [VDC] -> Saturation/1
  [ID] -> Gain2/1
  Gain1/1 -> Divide/1
  Demux2/3 -> Terminator1/1
  PID Controller2/1 -> Sum6/1
  PID Controller1/1 -> Gain4/1
  Divide1/1 -> Mux/2
  Gain4/1 -> Sum5/1
  Sum1/1 -> PID Controller3/1
  Selector/1 -> Sum/1
  Saturation1/1 -> Divide1/2
  [wt] -> dq0 to abc/2
  PID Controller/1 -> Integrator/1
  Demux1/3 -> Terminator/1
  Integrator/1 -> [wt], Alpha-Beta-Zero to dq1/2
  Constant2/1 -> Sum/2
  Sum/1 -> PID Controller/1
  abc to Alpha-Beta-Zero/1 -> [alphabeta], Alpha-Beta-Zero to dq0/1
  Divide/1 -> Mux/1
  dq0 to abc/1 -> Vabc/1, Scope6/1
  Gain/1 -> Sum6/2
  Demux1/1 -> [VD]
  Alpha-Beta-Zero to dq0/1 -> Demux1/1
  [VQ] -> Sum3/2
  Sum6/1 -> Sum7/1
  [VDC] -> Saturation1/1
  Alpha-Beta-Zero to dq1/1 -> Selector/1
  Sum7/1 -> Gain1/1
  [VD] -> Sum7/2
  [IQ] -> Sum1/2
  abc to dq0/1 -> Demux2/1
  [IQ] -> Gain/1
  Constant5/1 -> Sum1/1
  Saturation/1 -> Divide/2
  Demux2/1 -> [ID]
  Sum3/1 -> Gain3/1
  [wt] -> Alpha-Beta-Zero to dq0/2
  [Iabc] -> abc to dq0/1
  [wt] -> abc to dq0/2
  Gain2/1 -> Sum2/2
  Gain3/1 -> Divide1/1
  Constant4/1 -> Mux/3
  Demux2/2 -> [IQ]
  [ID] -> Sum5/2
  [IQ] -> Scope5/1
  [Vabc] -> abc to Alpha-Beta-Zero/1
  [VDC] -> Sum4/2

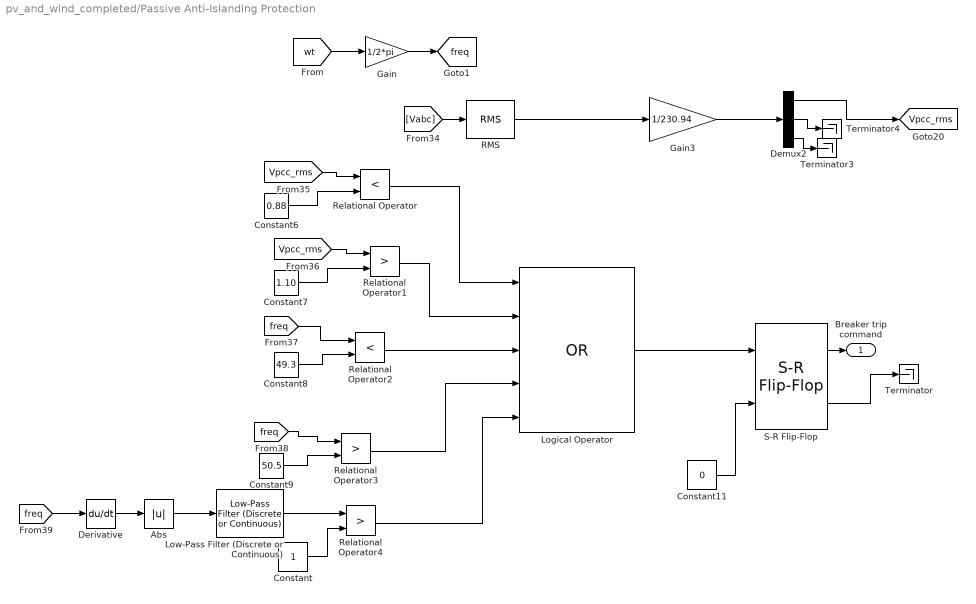
== system pv_and_wind_completed/Passive Anti-Islanding Protection ==
  Abs : Abs
  Constant : Constant
  Constant11 : Constant  Value=0  VectorParams1D=off  OutDataTypeStr=boolean
  Constant6 : Constant  Value=0.88
  Constant7 : Constant  Value=1.10
  Constant8 : Constant  Value=49.3
  Constant9 : Constant  Value=50.5
  Demux2 : Demux  Outputs=3
  Derivative : Derivative
  Gain : Gain  Gain=1/2*pi
  Gain3 : Gain  Gain=1/230.94
  Logical Operator : Logic  Operator=OR  Inputs=5  AllPortsSameDT=off  OutDataTypeStr=boolean
  Low-Pass Filter (Discrete or Continuous) : peGeneralControl/Low-Pass Filter (Discrete or Continuous)  K=1  T=1/(2*pi*10)  B=inf  A=-inf  Ts=-1
  RMS : powerlib_meascontrol/Measurements/RMS  TrueRMS=on  Freq=50  RMSInit=120  Ts=0
  Relational Operator : RelationalOperator  Operator=<  OutDataTypeStr=boolean  RndMeth=Simplest
  Relational Operator1 : RelationalOperator  Operator=>  OutDataTypeStr=boolean  RndMeth=Simplest
  Relational Operator2 : RelationalOperator  Operator=<  OutDataTypeStr=boolean  RndMeth=Simplest
  Relational Operator3 : RelationalOperator  Operator=>  OutDataTypeStr=boolean  RndMeth=Simplest
  Relational Operator4 : RelationalOperator  Operator=>  OutDataTypeStr=boolean  RndMeth=Simplest
  S-R Flip-Flop : simulink_extras/Flip Flops/S-R Flip-Flop  initial_condition=0
  Terminator : Terminator
  Terminator3 : Terminator
  Terminator4 : Terminator
  "Breaker trip command " : Outport
  tag scope: Vpcc_rms=global, freq=global
  wires:
  RMS/1 -> Gain3/1
  Constant6/1 -> Relational Operator/2
  Constant7/1 -> Relational Operator1/2
  [freq] -> Derivative/1
  Abs/1 -> Low-Pass Filter (Discrete or Continuous)/1
  [Vpcc_rms] -> Relational Operator1/1
  Gain3/1 -> Demux2/1
  [Vabc] -> RMS/1
  [freq] -> Relational Operator3/1
  Derivative/1 -> Abs/1
  Low-Pass Filter (Discrete or Continuous)/1 -> Relational Operator4/1
  Constant11/1 -> S-R Flip-Flop/2
  Logical Operator/1 -> S-R Flip-Flop/1
  Demux2/1 -> [Vpcc_rms]
  Constant8/1 -> Relational Operator2/2
  Constant/1 -> Relational Operator4/2
  Constant9/1 -> Relational Operator3/2
  [Vpcc_rms] -> Relational Operator/1
  Gain/1 -> [freq]
  Demux2/2 -> Terminator4/1
  Relational Operator1/1 -> Logical Operator/2
  Demux2/3 -> Terminator3/1
  Relational Operator3/1 -> Logical Operator/4
  Relational Operator/1 -> Logical Operator/1
  S-R Flip-Flop/2 -> Terminator/1
  Relational Operator2/1 -> Logical Operator/3
  [freq] -> Relational Operator2/1
  Relational Operator4/1 -> Logical Operator/5
  S-R Flip-Flop/1 -> "Breaker trip command "/1
  [wt] -> Gain/1

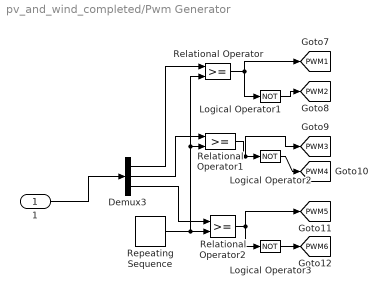
== system pv_and_wind_completed/Pwm Generator  ==
  1 : Inport
  Demux3 : Demux  Outputs=3
  Logical Operator1 : Logic  Operator=NOT  AllPortsSameDT=off  OutDataTypeStr=boolean
  Logical Operator2 : Logic  Operator=NOT  AllPortsSameDT=off  OutDataTypeStr=boolean
  Logical Operator3 : Logic  Operator=NOT  AllPortsSameDT=off  OutDataTypeStr=boolean
  Relational Operator : RelationalOperator  OutDataTypeStr=boolean  RndMeth=Simplest
  Relational Operator1 : RelationalOperator  OutDataTypeStr=boolean  RndMeth=Simplest
  Relational Operator2 : RelationalOperator  OutDataTypeStr=boolean  RndMeth=Simplest
  Repeating Sequence : simulink/Sources/Repeating Sequence  rep_seq_t=[0 0.00005 0.0001]  rep_seq_y=[-1 1 -1]
  tag scope: PWM1=global, PWM2=global, PWM3=global, PWM4=global, PWM5=global, PWM6=global
  wires:
  Relational Operator/1 -> Logical Operator1/1, [PWM1]
  Demux3/2 -> Relational Operator1/1
  Demux3/1 -> Relational Operator/1
  Relational Operator1/1 -> [PWM3], Logical Operator2/1
  Repeating Sequence/1 -> Relational Operator1/2, Relational Operator/2, Relational Operator2/2
  Demux3/3 -> Relational Operator2/1
  1/1 -> Demux3/1
  Relational Operator2/1 -> [PWM5], Logical Operator3/1
  Logical Operator1/1 -> [PWM2]
  Logical Operator2/1 -> [PWM4]
  Logical Operator3/1 -> [PWM6]

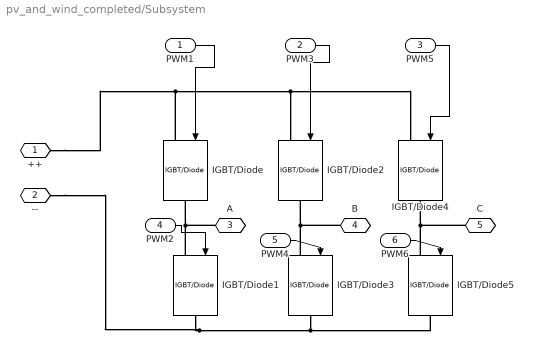
== system pv_and_wind_completed/Subsystem ==
  PWM1 : Inport
  PWM3 : Inport  Port=2
  PWM5 : Inport  Port=3
  PWM2 : Inport  Port=4
  PWM4 : Inport  Port=5
  PWM6 : Inport  Port=6
  IGBT/Diode{,1..5} (6 alike) : powerlib/Power Electronics/IGBT//Diode  Ron=1e-3  Rs=1e5  Cs=inf  Measurements=off
  ++ : PMIOPort  Side=Left
  -- : PMIOPort  Port=2  Side=Left
  A : PMIOPort  Port=3  Side=Right
  B : PMIOPort  Port=4  Side=Right
  C : PMIOPort  Port=5  Side=Right
  wires:
  PWM1/1 -> IGBT/Diode/1
  PWM4/1 -> IGBT/Diode3/1
  PWM6/1 -> IGBT/Diode5/1
  PWM3/1 -> IGBT/Diode2/1
  PWM5/1 -> IGBT/Diode4/1
  PWM2/1 -> IGBT/Diode1/1
  connections:
  IGBT/Diode1/RConn1 -- --/RConn1 -- IGBT/Diode3/RConn1 -- IGBT/Diode5/RConn1
  IGBT/Diode3/LConn1 -- B/RConn1 -- IGBT/Diode2/RConn1
  IGBT/Diode1/LConn1 -- A/RConn1 -- IGBT/Diode/RConn1
  IGBT/Diode5/LConn1 -- C/RConn1 -- IGBT/Diode4/RConn1
  IGBT/Diode/LConn1 -- ++/RConn1 -- IGBT/Diode2/LConn1 -- IGBT/Diode4/LConn1

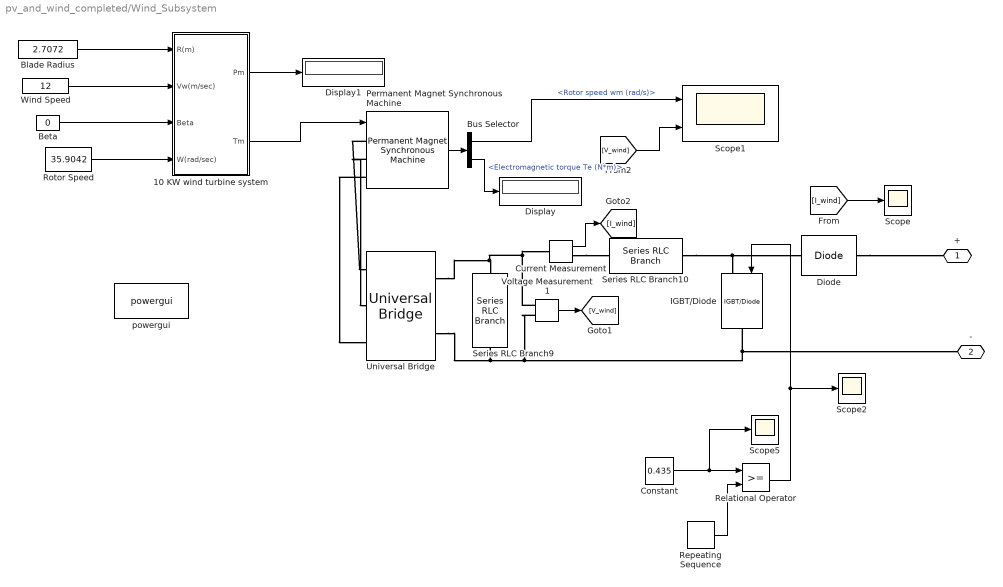
== system pv_and_wind_completed/Wind_Subsystem ==
  10 KW wind turbine system : Subsystem
  Beta : Constant  Value=0
  Blade Radius : Constant  Value=2.7072
  Bus Selector : BusSelector  OutputSignals=Rotor speed wm (rad/s),Electromagnetic torque Te (N*m)
  Constant : Constant  Value=0.435
  Current Measurement : powerlib/Measurements/Current Measurement  PhasorSimulation=off  OutputType=Complex  PSBequivalent=0
  Diode : powerlib/Power Electronics/Diode  Ron=0.001  Lon=0  Vf=0.8  IC=0  UseSnubber=0  Rs=500  Cs=250e-9  Measurements=off
  Display : Display
  Display1 : Display
  IGBT/Diode : powerlib/Power Electronics/IGBT//Diode  Ron=0.001  Rs=100  Cs=1e-6  Measurements=off
  Permanent Magnet Synchronous Machine : powerlib/Machines/Permanent Magnet Synchronous Machine  NbPhases=3  FluxDistribution=Sinusoidal  RotorType=Round  MechanicalLoad=Torque Tm  PresetModel=No  ShowDetailedParameters=on  MeasurementBus=off  Resistance=0.05486  Inductance=8.5e-3  dqInductances=[8.5e-3,8.5e-3]  La=0.000835  MachineConstant=Flux linkage established by magnets (V.s)  Flux=0.9  VoltageCst=326.4839  TorqueCst=2.7  Flat=120  Mechanical=[300 0.008 2 0]  PolePairs=4  InitialConditions=[157.08,0,0,0]  InitialConditions5ph=[0 0 0 0 0 0]  TsPowergui=0  TsBlock=-1  RefAngle=90 degrees behind phase A axis (modified Park)
      settings: SourceProductName=Simscape Power Systems
  Relational Operator : RelationalOperator  OutDataTypeStr=boolean  RndMeth=Simplest
  Repeating Sequence : simulink/Sources/Repeating Sequence  rep_seq_t="[0  0.0001]"  rep_seq_y=[0 1]
  Rotor Speed : Constant  Value=35.9042
  Scope : Scope
  Scope1 : Scope  NumInputPorts=2
  Scope2 : Scope
  Scope5 : Scope
  Series RLC Branch10 : powerlib/Elements/Series RLC Branch  LConnTagsString=__new0  RConnTagsString=__new0  BranchType=L  Resistance=2.3e-3  Inductance=10e-3  SetiL0=off  InitialCurrent=0  Capacitance=1e-6  Setx0=off  InitialVoltage=0  Measurements=None
  Series RLC Branch9 : powerlib/Elements/Series RLC Branch  LConnTagsString=__new0  RConnTagsString=__new0  BranchType=C  Resistance=1  Inductance=1e-3  SetiL0=off  InitialCurrent=0  Capacitance=2200e-6  Setx0=off  InitialVoltage=0  Measurements=None
  Universal Bridge : powerlib/Power Electronics/Universal Bridge  Arms=3  SnubberResistance=5000  SnubberCapacitance=inf  Device=Diodes  Ron=0.001  Lon=0  ForwardVoltages="[  0  0  ]"  ForwardVoltage=0  GTOparameters=[ 10e-6 , 20e-6 ]  IGBTparameters=[ 1e-6 , 2e-6 ]  Measurements=None  Measurements_2=None  converterType=Rectifier
  Voltage Measurement1 : powerlib/Measurements/Voltage Measurement  PhasorSimulation=off  OutputType=Complex  PSBequivalent=0
  Wind Speed : Constant  Value=12
  powergui : powerlib/powergui  Priority=1  SimulationMode=Discrete  SampleTime=1e-6  frequency=60  Iterations=50  frequencyindice=0  Pbase=100e6  ErrMax=1e-4  UnitsV=kV  UnitsW=MW  buscounter=0  FunctionMessages=off  echomessages=off  EnableUseOfTLC=off  CurrentSourceSwitches=off  DisableSnubberDevices=off  DisableRonSwitches=off  DisableVfSwitches=off  DisplayEquations=off  SolverType=Tustin/Backward Euler (TBE)  Interpol=off  ExternalGateDelay=off  methode=off  Ts=100  x0status=blocks  SPID=off  SwTol=0  HookPort=off  RestoreLinks=warning  ResistiveCurrentMeasurement=off  Frange=[0:2:500]  Ylog=off  Xlog=on  ShowGrid=off  save=off  variable=ZData  structure=0  ZoomFFT=off  StartTime=0.0  cycles=1  DisplayStyle=1  fundamental=60  FreqAxis=off  MaxFrequency=1000  frequencyindicesteady=1  RmsSteady=1  display=off
  + : PMIOPort  Side=Right
  - : PMIOPort  Port=2  Side=Right
  wires:
  Bus Selector/1 -> Scope1/1  "<Rotor speed wm (rad/s)>"
  [V_wind] -> Scope1/2
  Repeating Sequence/1 -> Relational Operator/2
  Permanent Magnet Synchronous Machine/1 -> Bus Selector/1
  Bus Selector/2 -> Display/1  "<Electromagnetic torque Te (N*m)>"
  Voltage Measurement1/1 -> [V_wind]
  Current Measurement/1 -> [I_wind]
  Constant/1 -> Relational Operator/1, Scope5/1
  Relational Operator/1 -> Scope2/1, IGBT/Diode/1
  Beta/1 -> 10 KW wind turbine system/3(Beta)
  Blade Radius/1 -> 10 KW wind turbine system/1(R(m))
  10 KW wind turbine system/1(Pm) -> Display1/1
  Wind Speed/1 -> 10 KW wind turbine system/2(Vw(m/sec))
  10 KW wind turbine system/2(Tm) -> Permanent Magnet Synchronous Machine/1
  Rotor Speed/1 -> 10 KW wind turbine system/4(W(rad/sec))
  [I_wind] -> Scope/1
  connections:
  Series RLC Branch9/LConn1 -- Universal Bridge/RConn1 -- Voltage Measurement1/LConn1 -- Current Measurement/LConn1
  IGBT/Diode/RConn1 -- Voltage Measurement1/LConn2 -- Universal Bridge/RConn2 -- Series RLC Branch9/RConn1 -- -/RConn1
  Series RLC Branch10/RConn1 -- Diode/LConn1 -- IGBT/Diode/LConn1
  Diode/RConn1 -- +/RConn1
  Permanent Magnet Synchronous Machine/LConn2 -- Universal Bridge/LConn2
  Permanent Magnet Synchronous Machine/LConn1 -- Universal Bridge/LConn1
  Current Measurement/RConn1 -- Series RLC Branch10/LConn1
  Permanent Magnet Synchronous Machine/LConn3 -- Universal Bridge/LConn3

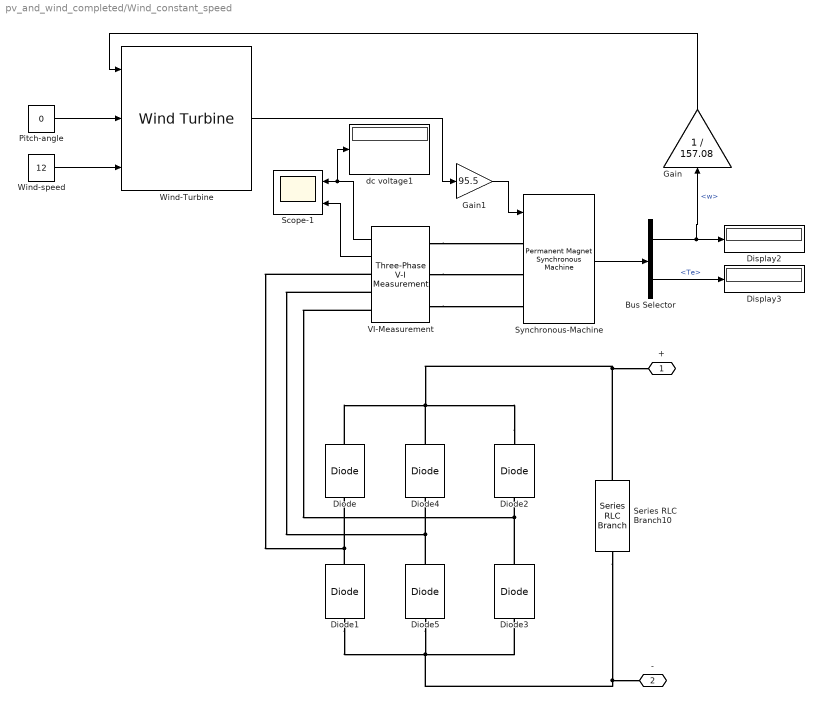
== system pv_and_wind_completed/Wind_constant_speed  ==
  " Synchronous-Machine" : powerlib/Machines/Permanent Magnet Synchronous Machine  NbPhases=3  FluxDistribution=Sinusoidal  RotorType=Round  MechanicalLoad=Torque Tm  PresetModel=No  ShowDetailedParameters=on  MeasurementBus=on  Resistance=0.0485  Inductance=8.5e-3  dqInductances=[8.5e-3,8.5e-3]  La=0.000395  MachineConstant=Flux linkage established by magnets (V.s)  Flux=0.1194  VoltageCst=86.6271  TorqueCst=0.7164  Flat=120  Mechanical=[0.0027 0.0004924 4 0]  PolePairs=4  InitialConditions=[0,0, 0,0]  InitialConditions5ph=[0 0 0 0 0 0]  TsPowergui=0  TsBlock=-1  RefAngle=90 degrees behind phase A axis (modified Park)
      link override From: GotoTag=T34_3314_1928570057647
      settings: SourceProductName=Simscape Power Systems
  " VI-Measurement" : powerlib/Measurements/Three-Phase V-I Measurement  VoltageMeasurement=phase-to-phase  SetLabelV=off  LabelV=Vabc  Vpu=off  VpuLL=off  CurrentMeasurement=yes  SetLabelI=off  LabelI=Iabc  Ipu=off  Pbase=100e6  Vbase=500e3  OutputType=Complex  PhasorSimulation=off  PSBequivalent=0
  Bus Selector : BusSelector  OutputSignals=w,Te
  Diode{,1..5} (6 alike) : powerlib/Power Electronics/Diode  Ron=0.001  Lon=0  Vf=0.8  IC=0  UseSnubber=0  Rs=500  Cs=250e-9  Measurements=off
  Display2 : Display
  Display3 : Display
  Gain : Gain  Gain=1 / 157.08
  Gain1 : Gain  Gain=95.5
  Pitch-angle : Constant  Value=0
  Scope-1 : Scope  NumInputPorts=2
  Series RLC Branch10 : powerlib/Elements/Series RLC Branch  LConnTagsString=__new0  RConnTagsString=__new0  BranchType=C  Resistance=1  Inductance=1e-3  SetiL0=off  InitialCurrent=0  Capacitance=10e-3  Setx0=off  InitialVoltage=0  Measurements=None
  Wind-Turbine : re_lib/Wind Generation/Wind Turbine  Pnom=1.5e6  Pelec_base=1.5e6/0.9  wind_base=12  P_wind_base=0.73  speed_nom=1.2  pitch_angle=2  c1_c6="[0.51763          116          0.4            5           21     0.006795]"  cp_nom=0.48  lambda_nom=8.1
      settings: SourceProductName=Simscape Power Systems  SourceProductBaseCode=PS
  Wind-speed : Constant  Value=12
  dc voltage1 : Display
  + : PMIOPort  Side=Left
  - : PMIOPort  Port=2  Side=Left
  wires:
  Wind-speed/1 -> Wind-Turbine/3
  " Synchronous-Machine"/1 -> Bus Selector/1
  Gain1/1 -> " Synchronous-Machine"/1
  " VI-Measurement"/1 -> dc voltage1/1, Scope-1/1
  Bus Selector/1 -> Gain/1, Display2/1  "<w>"
  Pitch-angle/1 -> Wind-Turbine/2
  Bus Selector/2 -> Display3/1  "<Te>"
  " VI-Measurement"/2 -> Scope-1/2
  Gain/1 -> Wind-Turbine/1
  Wind-Turbine/1 -> Gain1/1
  connections:
  " VI-Measurement"/RConn1 -- Diode/LConn1 -- Diode1/RConn1
  Diode5/LConn1 -- Series RLC Branch10/RConn1 -- -/RConn1 -- Diode1/LConn1 -- Diode3/LConn1
  Diode5/RConn1 -- Diode4/LConn1 -- " VI-Measurement"/RConn2
  Diode3/RConn1 -- " VI-Measurement"/RConn3 -- Diode2/LConn1
  Diode2/RConn1 -- Series RLC Branch10/LConn1 -- +/RConn1 -- Diode4/RConn1 -- Diode/RConn1
  " VI-Measurement"/LConn3 -- " Synchronous-Machine"/LConn3
  " VI-Measurement"/LConn1 -- " Synchronous-Machine"/LConn1
  " VI-Measurement"/LConn2 -- " Synchronous-Machine"/LConn2

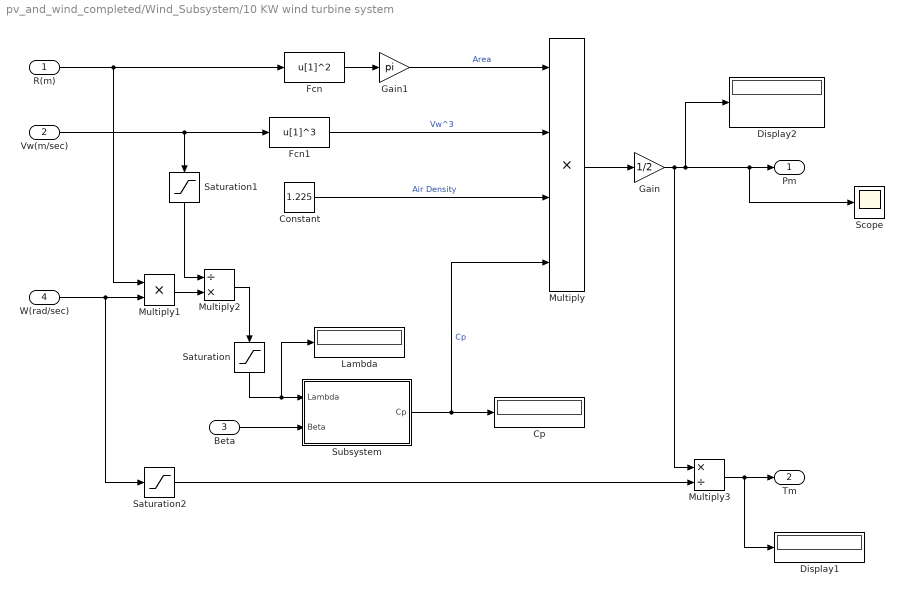
== system pv_and_wind_completed/Wind_Subsystem/10 KW wind turbine system ==
  R(m) : Inport
  Vw(m/sec) : Inport  Port=2
  Beta : Inport  Port=3
  W(rad/sec) : Inport  Port=4
  Constant : Constant  Value=1.225
  Cp : Display
  Display1 : Display
  Display2 : Display
  Fcn : Fcn  Expr=u[1]^2
  Fcn1 : Fcn  Expr=u[1]^3
  Gain : Gain  Gain=1/2
  Gain1 : Gain  Gain=pi
  Lambda : Display
  Multiply : Product  Inputs=4
  Multiply1 : Product
  Multiply2 : Product  Inputs=/*
  Multiply3 : Product  Inputs=*/
  Saturation : Saturate  UpperLimit=inf  LowerLimit=1e-6
  Saturation1 : Saturate  UpperLimit=inf  LowerLimit=1e-6
  Saturation2 : Saturate  UpperLimit=inf  LowerLimit=1e-6
  Scope : Scope
  Subsystem : Subsystem
  Pm : Outport
  Tm : Outport  Port=2
  wires:
  Gain/1 -> Multiply3/1, Display2/1, Scope/1, Pm/1
  Multiply/1 -> Gain/1
  Gain1/1 -> Multiply/1  "Area"
  Fcn1/1 -> Multiply/2  "Vw^3"
  Constant/1 -> Multiply/3  "Air Density"
  Subsystem/1(Cp) -> Cp/1, Multiply/4  "Cp"
  Fcn/1 -> Gain1/1
  R(m)/1 -> Multiply1/1, Fcn/1
  Vw(m/sec)/1 -> Fcn1/1, Saturation1/1
  Beta/1 -> Subsystem/2(Beta)
  W(rad/sec)/1 -> Saturation2/1, Multiply1/2
  Multiply1/1 -> Multiply2/2
  Multiply2/1 -> Saturation/1
  Saturation1/1 -> Multiply2/1
  Saturation2/1 -> Multiply3/2
  Multiply3/1 -> Display1/1, Tm/1
  Saturation/1 -> Lambda/1, Subsystem/1(Lambda)

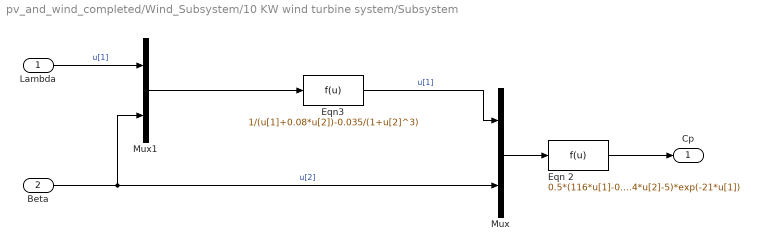
== system pv_and_wind_completed/Wind_Subsystem/10 KW wind turbine system/Subsystem ==
  Lambda : Inport
  Beta : Inport  Port=2
  Eqn 2 : Fcn  Expr=0.5*(116*u[1]-0.4*u[2]-5)*exp(-21*u[1])
  Eqn3 : Fcn  Expr=1/(u[1]+0.08*u[2])-0.035/(1+u[2]^3)
  Mux : Mux  Inputs=2
  Mux1 : Mux  Inputs=2
  Cp : Outport
  wires:
  Eqn 2/1 -> Cp/1
  Mux/1 -> Eqn 2/1
  Lambda/1 -> Mux1/1  "u[1]"
  Eqn3/1 -> Mux/1  "u[1]"
  Beta/1 -> Mux1/2, Mux/2  "u[2]"
  Mux1/1 -> Eqn3/1

== matlab function pv_and_wind_completed/MATLAB Function ==
  data: t input; G output; T output
function [G, T] = solar_profile_24h(t)
% Compresses a 24-hour irradiance/temperature profile into 2.4s of sim time
% Scale: 0.1 sim-second = 1 real hour (2.4s total = 24 hours)

    % --- Convert sim time to hour-of-day ---
    t_hr = t / 0.1;   % equivalent to t * 10

    % --- Irradiance profile (representative clear-sky day) ---
    sunrise = 6;       % 6:00 AM
    sunset  = 18;       % 6:00 PM
    Gmax    = 1000;     % peak irradiance, W/m^2 (STC-consistent)

    if t_hr >= sunrise && t_hr <= sunset
        G = Gmax * sin(pi * (t_hr - sunrise) / (sunset - sunrise));
    else
        G = 0;
    end
    G = max(G, 0);

    % --- Ambient temperature profile ---
    Tmean = 23.5;      % deg C, daily average
    Tamp  = 8.5;       % deg C, swing above/below mean
    T = Tmean + Tamp * sin(2*pi*(t_hr - 9) / 24);

end

== matlab function pv_and_wind_completed/DC-DC Boost Converter with MPPT/MPPT ==
  data: V input; Vref output; I input

function Vref = MPPT(V,I)

Vrefmax = 50;
Vrefmin = 0;
Vrefinit = 45;
deltaVref = 1;
persistent Vold Pold Vrefold;

dataType = 'double';

if isempty(Vold)
    Vold = 0;
    Pold = 0;
    Vrefold = Vrefinit;
end

P = V*I;
dV = V-Vold;
dP = P-Pold;

if dP ~= 0
    if dP<0
        if dV<0
         Vref = Vrefold + deltaVref;
        else
            Vref = Vrefold - deltaVref;
        end
    else
        if dV<0
            Vref = Vrefold - deltaVref;
        else
            Vref = Vrefold + deltaVref;
        end
    end
else 
     Vref = Vrefold;
end

if Vref >= Vrefmax || Vref <= Vrefmin
    Vref = Vrefold;
end

Vrefold = Vref;
Vold = V;
Pold = P;
